simulink model "kerekszimulacio"  (R2018a)
settings: Solver=FixedStepDiscrete  StartTime=0.0  StopTime=50000  RelTol=1e-3
libraries: xbsIndex_r4 x19, simulink x2
settings Model: Creator=peter  LastModifiedBy=peter

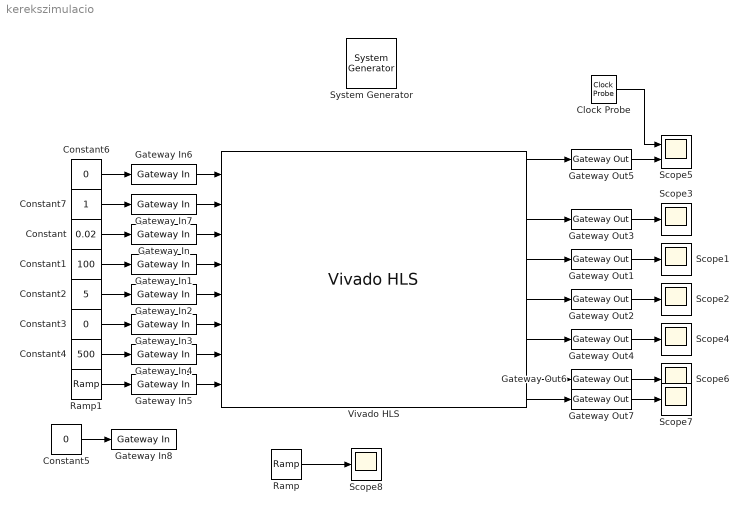
== system kerekszimulacio ==
  " System Generator" : xbsIndex_r4/ System Generator  Tag=genX  xilinxfamily=kintex7  part=xc7k325t  speed=-2  package=ffg900  synthesis_tool=Vivado  clock_wrapper=Clock Enables  directory=./netlist  proj_type=Vivado  Synth_file=Vivado Synthesis Defaults  Impl_file=Vivado Implementation Defaults  testbench=off  simulink_period=1  sysclk_period=10  dcm_input_clock_period=10  incr_netlist=off  trim_vbits=Everywhere in SubSystem  dbl_ovrd=According to Block Masks  core_generation=According to Block Masks  run_coregen=off  deprecated_control=off  eval_field=0  block_type=sysgen
  Clock Probe : xbsIndex_r4/Clock Probe  block_type=clkprobe
      settings: infoedit="Clock probe.  Produces an output of type double that mirrors the hardware system clock.<br><br>Hardware notes:  This block is ignored when hardware is generated."
  Constant : Constant  Value=0.02
  Constant1 : Constant  Value=100
  Constant2 : Constant  Value=5
  Constant3 : Constant  Value=0
  Constant4 : Constant  Value=500
  Constant5 : Constant  Value=0
  Constant6 : Constant  Value=0
  Constant7 : Constant
  Gateway In{,1..5,8} (7 alike) : xbsIndex_r4/Gateway In  gui_display_data_type=Floating-point  arith_type=Floating-point  n_bits=16  bin_pt=14  preci_type=Single  exp_width=8  frac_width=24  rows=1  columns=1  quantization="Round  (unbiased: +/- Inf)"  overflow=Saturate  period=1  UseAsADC=off  ADCChannel='1'  interface=None  automatic_assignment=on  address_offset=hex2dec('00')  intf_name=''  intf_description=''  default_value=0  timing_constraint=None  locs_specified=off  LOCs={}  io_standard={}  inherit_from_input=off  hdl_port=on  dbl_ovrd=off  block_type=gatewayin
  Gateway In6 : xbsIndex_r4/Gateway In  gui_display_data_type=Boolean  arith_type=Boolean  n_bits=16  bin_pt=14  preci_type=Single  exp_width=8  frac_width=24  rows=1  columns=1  quantization="Round  (unbiased: +/- Inf)"  overflow=Saturate  period=1  UseAsADC=off  ADCChannel='1'  interface=None  automatic_assignment=on  address_offset=hex2dec('00')  intf_name=''  intf_description=''  default_value=0  timing_constraint=None  locs_specified=off  LOCs={}  io_standard={}  inherit_from_input=off  hdl_port=on  dbl_ovrd=off  block_type=gatewayin
  Gateway In7 : xbsIndex_r4/Gateway In  gui_display_data_type=Boolean  arith_type=Boolean  n_bits=16  bin_pt=14  preci_type=Single  exp_width=8  frac_width=24  rows=1  columns=1  quantization="Round  (unbiased: +/- Inf)"  overflow=Saturate  period=1  UseAsADC=off  ADCChannel='1'  interface=None  automatic_assignment=on  address_offset=hex2dec('00')  intf_name=''  intf_description=''  default_value=0  timing_constraint=None  locs_specified=off  LOCs={}  io_standard={}  inherit_from_input=off  hdl_port=on  dbl_ovrd=off  block_type=gatewayin
  Gateway Out{1..7} (7 alike) : xbsIndex_r4/Gateway Out  inherit_from_input=off  hdl_port=on  rows=1  columns=1  UseAsDAC=off  DACChannel='1'  interface=None  automatic_assignment=on  address_offset=hex2dec('00')  intf_name=''  intf_description=''  timing_constraint=None  locs_specified=off  LOCs={}  io_standard={}  block_type=gatewayout
  Ramp : simulink/Sources/Ramp  slope=0.000005  start=30000  InitialOutput=0
  Ramp1 : simulink/Sources/Ramp  slope=0.000005  start=30000  InitialOutput=0
  Scope{1..4,6..8} (7 alike) : Scope
  Scope5 : Scope  NumInputPorts=2
  Vivado HLS : xbsIndex_r4/Vivado HLS  anytable='D:/Dev/Repos/CarSimOnFPGA/solution2'  fast_sim=off  display_datatype=on  rate_propagation_method=Simulink system period  model_file_path=''  latency=1  block_type=hls
      settings: infoedit=This block allows including C,C++ and SystemC source files in System Generator for DSP designs.
  wires:
  Gateway In/1 -> Vivado HLS/3
  Gateway In1/1 -> Vivado HLS/4
  Gateway In2/1 -> Vivado HLS/5
  Gateway In3/1 -> Vivado HLS/6
  Vivado HLS/6 -> Gateway Out1/1
  Vivado HLS/8 -> Gateway Out2/1
  Ramp1/1 -> Gateway In5/1
  Constant4/1 -> Gateway In4/1
  Constant3/1 -> Gateway In3/1
  Constant2/1 -> Gateway In2/1
  Constant1/1 -> Gateway In1/1
  Constant/1 -> Gateway In/1
  Gateway Out2/1 -> Scope2/1
  Gateway Out1/1 -> Scope1/1
  Constant6/1 -> Gateway In6/1
  Constant7/1 -> Gateway In7/1
  Gateway In6/1 -> Vivado HLS/1
  Gateway In7/1 -> Vivado HLS/2
  Gateway Out5/1 -> Scope5/2
  Vivado HLS/1 -> Gateway Out5/1
  Gateway In4/1 -> Vivado HLS/7
  Clock Probe/1 -> Scope5/1
  Vivado HLS/4 -> Gateway Out3/1
  Gateway Out3/1 -> Scope3/1
  Vivado HLS/10 -> Gateway Out4/1
  Gateway Out4/1 -> Scope4/1
  Vivado HLS/12 -> Gateway Out6/1
  Gateway Out6/1 -> Scope6/1
  Gateway Out7/1 -> Scope7/1
  Vivado HLS/13 -> Gateway Out7/1
  Ramp/1 -> Scope8/1
  Constant5/1 -> Gateway In8/1
  Gateway In5/1 -> Vivado HLS/8
